simulink model "case2"  (R2022a)
settings: Solver=VariableStepAuto  StartTime=0.0  StopTime=40  RelTol=1e-3
undefined symbols (not defined in the file): c1, c2, k1, k2, m1, m2
settings Model: Creator=RISHI  LastModifiedBy=Z0150218

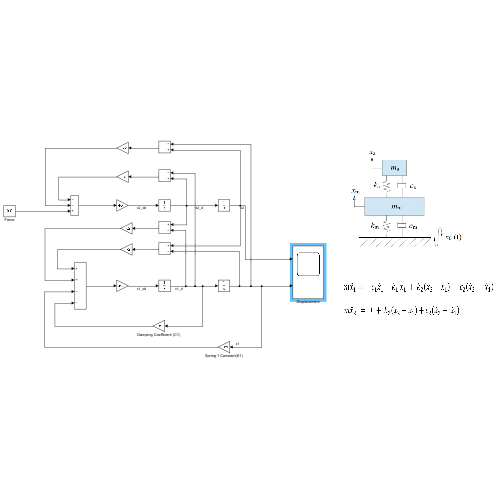
[thumbnail: Simulink's stored preview of the top-level diagram]
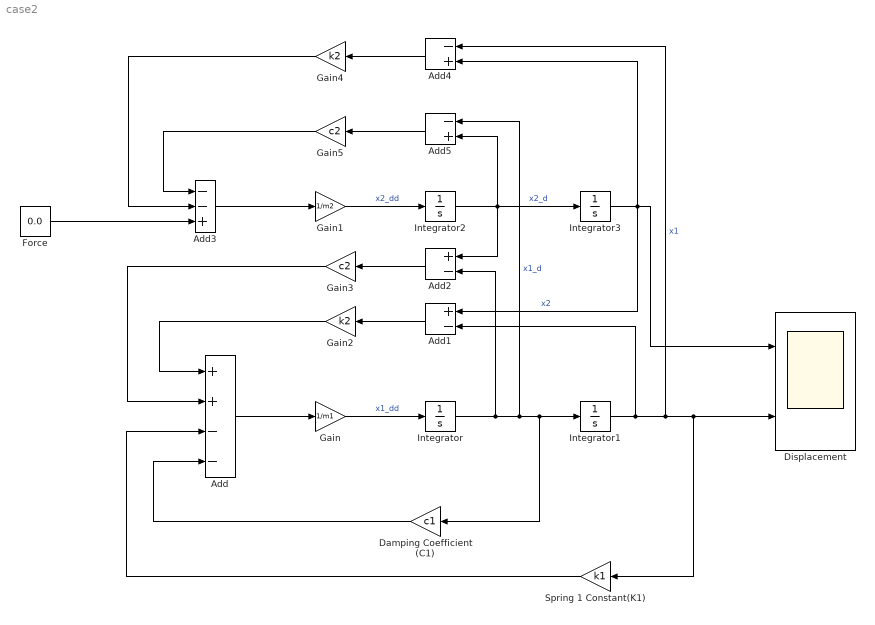
== system case2 ==
  Add : Sum  Inputs=++--
  Add1 : Sum  Inputs=+-
  Add2 : Sum  Inputs=+-
  Add3 : Sum  Inputs=--+
  Add4 : Sum  Inputs=-+
  Add5 : Sum  Inputs=-+
  Damping Coefficient (C1) : Gain  Gain=c1
  Displacement : Scope  NumInputPorts=2
  Force : Constant  Value=0.0
  Gain : Gain  Gain=1/m1
  Gain1 : Gain  Gain=1/m2
  Gain2 : Gain  Gain=k2
  Gain3 : Gain  Gain=c2
  Gain4 : Gain  Gain=k2
  Gain5 : Gain  Gain=c2
  Integrator : Integrator
  Integrator1 : Integrator  InitialCondition=2
  Integrator2 : Integrator
  Integrator3 : Integrator  InitialCondition=2
  Spring 1 Constant(K1) : Gain  Gain=k1
  wires:
  Integrator/1 -> Add5/1, Damping Coefficient (C1)/1, Integrator1/1, Add2/2  "x1_d"
  Gain/1 -> Integrator/1  "x1_dd"
  Integrator1/1 -> Add1/2, Add4/1, Spring 1 Constant(K1)/1, Displacement/2  "x1"
  Add/1 -> Gain/1
  Spring 1 Constant(K1)/1 -> Add/3
  Damping Coefficient (C1)/1 -> Add/4
  Integrator2/1 -> Add5/2, Add2/1, Integrator3/1  "x2_d"
  Gain1/1 -> Integrator2/1  "x2_dd"
  Integrator3/1 -> Add4/2, Add1/1, Displacement/1  "x2"
  Add3/1 -> Gain1/1
  Add1/1 -> Gain2/1
  Gain2/1 -> Add/1
  Add2/1 -> Gain3/1
  Gain3/1 -> Add/2
  Add4/1 -> Gain4/1
  Gain4/1 -> Add3/2
  Add5/1 -> Gain5/1
  Gain5/1 -> Add3/1
  Force/1 -> Add3/3
